simulink model "Motor_Control"  (R2020b)
settings: Solver=FixedStepAuto  StartTime=0.0  StopTime=10.0  RelTol=1e-3
settings Model: Creator=True  LastModifiedBy=True

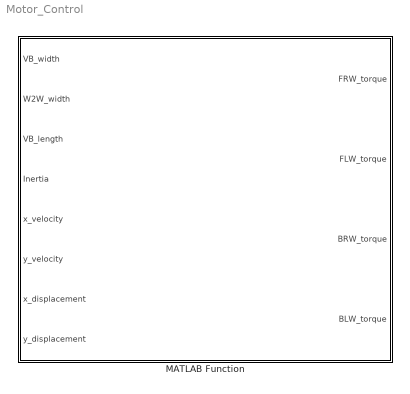
== system Motor_Control ==
  MATLAB Function : MATLAB Function  TreatAsAtomicUnit=on

== matlab function Motor_Control/MATLAB Function ==
  data: VB_width input; FRW_torque output; W2W_width input; VB_length input; Inertia input; x_velocity input; y_velocity input; x_displacement input; y_displacement input; FLW_torque output; BRW_torque output; BLW_torque output
function [FRW_torque,FLW_torque,BRW_torque,BLW_torque] = Motor_Control(VB_width,W2W_width,VB_length,Inertia,x_velocity,y_velocity,x_displacement,y_displacement)

ref_table = readmatrix("Track_dims.csv");
x_displacement_ar = ref_table(:,1);
y_displacement_ar = ref_table(:,2);
driving_radius_ar = ref_table(:,3);
target_velocity = 1;

driving_radius = driving_radius_ar((x_displacement_ar == x_displacement) & (y_displacement_ar == y_displacement));

velocity = (x_velocity^2 + y_velocity^2)^0.5;
angular_v = velocity / driving_radius;
angular_target = target_velocity / driving_radius;

theta_1 = atan((2*VB_length)/(2*driving_radius - VB_width));
theta_2 = atan((2*VB_length)/(2*driving_radius + VB_width));

radius_1 = (VB_length/sin(theta_1)) - ((W2W_width - VB_width)/2);
radius_2 = (VB_length/sin(theta_2)) + ((W2W_width - VB_width)/2);
radius_3 = (VB_length/tan(theta_1)) - ((W2W_width - VB_width)/2);
radius_4 = (VB_length/tan(theta_2)) + ((W2W_width - VB_width)/2);

if velocity < target_velocity
    if driving_radius > 0
        FRW_torque = Inertia * (angular_v^2) * radius_1;
        FLW_torque = Inertia * (angular_v^2) * radius_2;
        BRW_torque = Inertia * (angular_v^2) * radius_3;
        BLW_torque = Inertia * (angular_v^2) * radius_4;
    elseif driving_radius < 0
        FLW_torque = Inertia * (angular_v^2) * radius_1;
        FRW_torque = Inertia * (angular_v^2) * radius_2;
        BLW_torque = Inertia * (angular_v^2) * radius_3;
        BRW_torque = Inertia * (angular_v^2) * radius_4;
    else
        FRW_torque = Inertia * (angular_v^2) * driving_radius;
        FLW_torque = Inertia * (angular_v^2) * driving_radius;
        BRW_torque = Inertia * (angular_v^2) * driving_radius;
        BLW_torque = Inertia * (angular_v^2) * driving_radius;
    end
elseif velocity > target_velocity
    if driving_radius > 0
        FRW_torque = Inertia * (angular_target^2) * radius_1;
        FLW_torque = Inertia * (angular_target^2) * radius_2;
        BRW_torque = Inertia * (angular_target^2) * radius_3;
        BLW_torque = Inertia * (angular_target^2) * radius_4;
    elseif driving_radius < 0
        FLW_torque = Inertia * (angular_target^2) * radius_1;
        FRW_torque = Inertia * (angular_target^2) * radius_2;
        BLW_torque = Inertia * (angular_target^2) * radius_3;
        BRW_torque = Inertia * (angular_target^2) * radius_4;
    else
        FRW_torque = Inertia * (angular_target^2) * driving_radius;
        FLW_torque = Inertia * (angular_target^2) * driving_radius;
        BRW_torque = Inertia * (angular_target^2) * driving_radius;
        BLW_torque = Inertia * (angular_target^2) * driving_radius;
    end
else
    FRW_torque = 0;
    FLW_torque = 0;
    BRW_torque = 0;
    BLW_torque = 0;
end
